simulink model "RL_Circuit"  (R2022a)
settings: Solver=VariableStepAuto  StartTime=0.0  StopTime=10.0  RelTol=1e-3
undefined symbols (not defined in the file): E, L, R
settings Model: Creator=Adam Ghatta  LastModifiedBy=Adam Ghatta

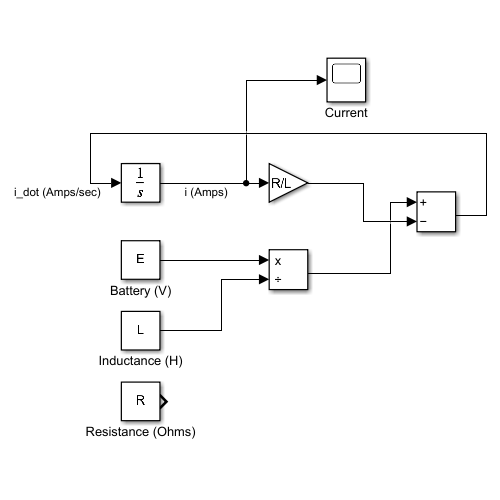
[thumbnail: Simulink's stored preview of the top-level diagram]
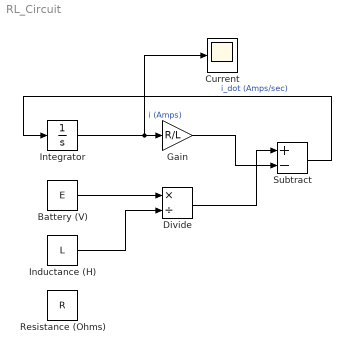
== system RL_Circuit ==
  Battery (V) : Constant  Value=E
  Current : Scope
  Divide : Product  Inputs=*/
  Gain : Gain  Gain=R/L
  Inductance (H) : Constant  Value=L
  Integrator : Integrator
  Resistance (Ohms) : Constant  Value=R
  Subtract : Sum  Inputs=+-
  wires:
  Integrator/1 -> Current/1, Gain/1  "i (Amps)"
  Subtract/1 -> Integrator/1  "i_dot (Amps/sec)"
  Battery (V)/1 -> Divide/1
  Inductance (H)/1 -> Divide/2
  Gain/1 -> Subtract/2
  Divide/1 -> Subtract/1
